simulink model "FG_costante_vs_filtro"  (R2020a)
settings: Solver=VariableStepAuto  StartTime=0.0  StopTime=10.0  RelTol=1e-3
values from neighbouring files (symbols this model uses):
  Aa = 2    [dati_tesi_modellosimulink.m]
  g = 9.81    [dati_tesi_modellosimulink.m]
  L = 0.3    [dati_tesi_modellosimulink.m]
  Lc = L/2    (= 0.15)    [dati_tesi_modellosimulink.m]
  M = 4    [dati_tesi_modellosimulink.m]
  mc = 0    [dati_tesi_modellosimulink.m]
  Ra = 1    [dati_tesi_modellosimulink.m]
  wb = 2*pi*2    (= 12.5663706144)    [dati_tesi_modellosimulink.m]
libraries: fuzblock x5, simulink x3, simulink_extras x2
settings Model: Creator=laura  LastModifiedBy=laura

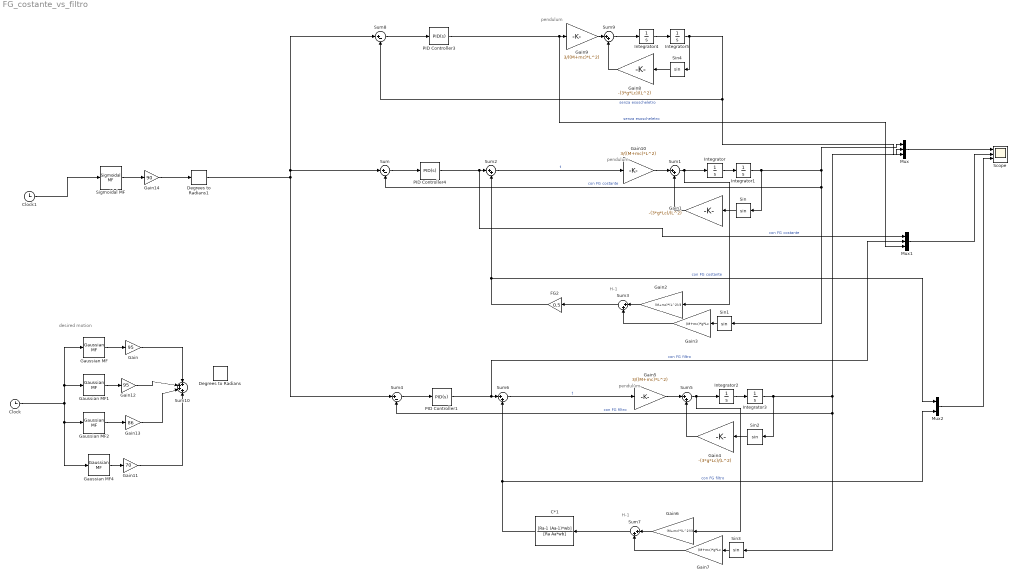
== system FG_costante_vs_filtro ==
  note: H-1
  note: pendulum
  note: pendulum
  note: H-1
  note: pendulum
  note: desired motion
  C*1 : TransferFcn  Numerator=[Ra-1 (Aa-1)*wb]  Denominator=[Ra Aa*wb]
  Clock : Clock
  Clock1 : Clock
  Degrees to Radians : simulink_extras/Transformations/Degrees to Radians
  Degrees to Radians1 : simulink_extras/Transformations/Degrees to Radians
  FG2 : Gain  Gain=0.5
  Gain : Gain  Gain=95
  Gain1 : Gain  Gain=-(3*g*Lc)/(L^2)
  Gain10 : Gain  Gain=3/((M+mc)*L^2)
  Gain11 : Gain  Gain=70
  Gain12 : Gain  Gain=95
  Gain13 : Gain  Gain=86
  Gain14 : Gain  Gain=90
  Gain2 : Gain  Gain=(M+mc)*(L^2)/3
  Gain3 : Gain  Gain=(M+mc)*g*Lc
  Gain4 : Gain  Gain=-(3*g*Lc)/(L^2)
  Gain5 : Gain  Gain=3/((M+mc)*L^2)
  Gain6 : Gain  Gain=(M+mc)*(L^2)/3
  Gain7 : Gain  Gain=(M+mc)*g*Lc
  Gain8 : Gain  Gain=-(3*g*Lc)/(L^2)
  Gain9 : Gain  Gain=3/((M+mc)*L^2)
  Gaussian MF : fuzblock/Membership  Functions/Gaussian MF  sigma=0.4  mu=1.78
      settings: SourceProductBaseCode=FL
  Gaussian MF1 : fuzblock/Membership  Functions/Gaussian MF  sigma=0.4  mu=7
      settings: SourceProductBaseCode=FL
  Gaussian MF2 : fuzblock/Membership  Functions/Gaussian MF  sigma=0.38  mu=3.42
      settings: SourceProductBaseCode=FL
  Gaussian MF4 : fuzblock/Membership  Functions/Gaussian MF  sigma=0.32  mu=2.63
      settings: SourceProductBaseCode=FL
  Integrator{,1..5} (6 alike) : Integrator
  Mux : Mux  Inputs=3
  Mux1 : Mux  Inputs=3
  Mux2 : Mux  Inputs=2
  PID Controller1 : simulink/Continuous/PID Controller  Controller=PID  Form=Parallel  TimeDomain=Continuous-time  UseExternalTs=off  SampleTime=-1  IntegratorMethod=Forward Euler  FilterMethod=Forward Euler  ControllerParametersSource=internal  P=20.396  I=105.7651  D=6.3413  UseFilter=on  N=150.7964  TunerSelectOption=Transfer Function Based (PID Tuner App)  InitialConditionSource=internal  InitialConditionForIntegrator=0  InitialConditionForFilter=0  DifferentiatorICPrevScaledInput=0  ExternalReset=none  TrackingMode=off  Kt=1  LimitOutput=off  UpperSaturationLimit=inf  LowerSaturationLimit=-inf  LinearizeAsGain=on  AntiWindupMode=none  Kb=1  POutMin=[]  POutMax=[]  IOutMin=[]  IOutMax=[]  DOutMin=[]  DOutMax=[]  NOutMin=[]  NOutMax=[]  SumOutMin=[]  SumOutMax=[]  SaturationOutMin=[]  SaturationOutMax=[]  PParamMin=[]  PParamMax=[]  IParamMin=[]  IParamMax=[]  DParamMin=[]  DParamMax=[]  NParamMin=[]  NParamMax=[]  KbParamMin=[]  KbParamMax=[]  KtParamMin=[]  KtParamMax=[]  KbOutMin=[]  KbOutMax=[]  KtOutMin=[]  KtOutMax=[]  IntegratorOutMin=[]  IntegratorOutMax=[]  FilterOutMin=[]  FilterOutMax=[]  SumI1OutMin=[]  SumI1OutMax=[]  SumI2OutMin=[]  SumI2OutMax=[]  SumI3OutMin=[]  SumI3OutMax=[]  SumI4OutMin=[]  SumI4OutMax=[]  SumDOutMin=[]  SumDOutMax=[]  DifferentiatorOutMin=[]  DifferentiatorOutMax=[]  FilterDiffOutCoefMin=[]  FilterDiffOutCoefMax=[]  ReciprocalOutMin=[]  ReciprocalOutMax=[]  SumDenOutMin=[]  SumDenOutMax=[]  SumNumOutMin=[]  SumNumOutMax=[]  DivideOutMin=[]  DivideOutMax=[]  UdiffTsProdOutMin=[]  UdiffTsProdOutMax=[]  NTsProdOutMin=[]  NTsProdOutMax=[]  UintegralTsProdOutMin=[]  UintegralTsProdOutMax=[]  UngainTsProdOutMin=[]  UngainTsProdOutMax=[]  IntegratorContinuousStateAttributes=''  IntegratorStateMustResolveToSignalObject=off  IntegratorRTWStateStorageClass=Auto  FilterContinuousStateAttributes=''  FilterStateMustResolveToSignalObject=off  FilterRTWStateStorageClass=Auto  ParallelPVariant=InternalParameters  IdealPVariant=Disabled  IVariant=InternalParameters  DVariant=InternalParameters  IntegratorVariant=Continuous  SatVariant=Disabled  AWVariant=Passthrough  PCopyVariant=Disabled  TRVariant=Disabled  FdbkBlocksVariant=Forward  IdealPFdbkVariant=Disabled  SatFdbkVariant=Disabled  DerivativeFilterVariant=ContFilter  NVariant=InternalParameters  NCopyVariant=Disabled  FilterICVariant=InternalICsFilter  IntegratorICVariant=InternalICs  ExternalResetVariant=Disabled  TRSumVariant=Passthrough  SumFdbkVariant=Disabled  SumVariant=Sum_PID  TsampFilterVariant=InternalTs  TsampNgainVariant=Passthrough  TsampIntegralVariant=Passthrough
  PID Controller3 : simulink/Continuous/PID Controller  Controller=PID  Form=Parallel  TimeDomain=Continuous-time  UseExternalTs=off  SampleTime=-1  IntegratorMethod=Forward Euler  FilterMethod=Forward Euler  ControllerParametersSource=internal  P=20.396  I=105.7651  D=6.3413  UseFilter=on  N=150.7964  TunerSelectOption=Transfer Function Based (PID Tuner App)  InitialConditionSource=internal  InitialConditionForIntegrator=0  InitialConditionForFilter=0  DifferentiatorICPrevScaledInput=0  ExternalReset=none  TrackingMode=off  Kt=1  LimitOutput=off  UpperSaturationLimit=inf  LowerSaturationLimit=-inf  LinearizeAsGain=on  AntiWindupMode=none  Kb=1  POutMin=[]  POutMax=[]  IOutMin=[]  IOutMax=[]  DOutMin=[]  DOutMax=[]  NOutMin=[]  NOutMax=[]  SumOutMin=[]  SumOutMax=[]  SaturationOutMin=[]  SaturationOutMax=[]  PParamMin=[]  PParamMax=[]  IParamMin=[]  IParamMax=[]  DParamMin=[]  DParamMax=[]  NParamMin=[]  NParamMax=[]  KbParamMin=[]  KbParamMax=[]  KtParamMin=[]  KtParamMax=[]  KbOutMin=[]  KbOutMax=[]  KtOutMin=[]  KtOutMax=[]  IntegratorOutMin=[]  IntegratorOutMax=[]  FilterOutMin=[]  FilterOutMax=[]  SumI1OutMin=[]  SumI1OutMax=[]  SumI2OutMin=[]  SumI2OutMax=[]  SumI3OutMin=[]  SumI3OutMax=[]  SumI4OutMin=[]  SumI4OutMax=[]  SumDOutMin=[]  SumDOutMax=[]  DifferentiatorOutMin=[]  DifferentiatorOutMax=[]  FilterDiffOutCoefMin=[]  FilterDiffOutCoefMax=[]  ReciprocalOutMin=[]  ReciprocalOutMax=[]  SumDenOutMin=[]  SumDenOutMax=[]  SumNumOutMin=[]  SumNumOutMax=[]  DivideOutMin=[]  DivideOutMax=[]  UdiffTsProdOutMin=[]  UdiffTsProdOutMax=[]  NTsProdOutMin=[]  NTsProdOutMax=[]  UintegralTsProdOutMin=[]  UintegralTsProdOutMax=[]  UngainTsProdOutMin=[]  UngainTsProdOutMax=[]  IntegratorContinuousStateAttributes=''  IntegratorStateMustResolveToSignalObject=off  IntegratorRTWStateStorageClass=Auto  FilterContinuousStateAttributes=''  FilterStateMustResolveToSignalObject=off  FilterRTWStateStorageClass=Auto  ParallelPVariant=InternalParameters  IdealPVariant=Disabled  IVariant=InternalParameters  DVariant=InternalParameters  IntegratorVariant=Continuous  SatVariant=Disabled  AWVariant=Passthrough  PCopyVariant=Disabled  TRVariant=Disabled  FdbkBlocksVariant=Forward  IdealPFdbkVariant=Disabled  SatFdbkVariant=Disabled  DerivativeFilterVariant=ContFilter  NVariant=InternalParameters  NCopyVariant=Disabled  FilterICVariant=InternalICsFilter  IntegratorICVariant=InternalICs  ExternalResetVariant=Disabled  TRSumVariant=Passthrough  SumFdbkVariant=Disabled  SumVariant=Sum_PID  TsampFilterVariant=InternalTs  TsampNgainVariant=Passthrough  TsampIntegralVariant=Passthrough
  PID Controller4 : simulink/Continuous/PID Controller  Controller=PID  Form=Parallel  TimeDomain=Continuous-time  UseExternalTs=off  SampleTime=-1  IntegratorMethod=Forward Euler  FilterMethod=Forward Euler  ControllerParametersSource=internal  P=20.396  I=105.7651  D=6.3413  UseFilter=on  N=150.7964  TunerSelectOption=Transfer Function Based (PID Tuner App)  InitialConditionSource=internal  InitialConditionForIntegrator=0  InitialConditionForFilter=0  DifferentiatorICPrevScaledInput=0  ExternalReset=none  TrackingMode=off  Kt=1  LimitOutput=off  UpperSaturationLimit=inf  LowerSaturationLimit=-inf  LinearizeAsGain=on  AntiWindupMode=none  Kb=1  POutMin=[]  POutMax=[]  IOutMin=[]  IOutMax=[]  DOutMin=[]  DOutMax=[]  NOutMin=[]  NOutMax=[]  SumOutMin=[]  SumOutMax=[]  SaturationOutMin=[]  SaturationOutMax=[]  PParamMin=[]  PParamMax=[]  IParamMin=[]  IParamMax=[]  DParamMin=[]  DParamMax=[]  NParamMin=[]  NParamMax=[]  KbParamMin=[]  KbParamMax=[]  KtParamMin=[]  KtParamMax=[]  KbOutMin=[]  KbOutMax=[]  KtOutMin=[]  KtOutMax=[]  IntegratorOutMin=[]  IntegratorOutMax=[]  FilterOutMin=[]  FilterOutMax=[]  SumI1OutMin=[]  SumI1OutMax=[]  SumI2OutMin=[]  SumI2OutMax=[]  SumI3OutMin=[]  SumI3OutMax=[]  SumI4OutMin=[]  SumI4OutMax=[]  SumDOutMin=[]  SumDOutMax=[]  DifferentiatorOutMin=[]  DifferentiatorOutMax=[]  FilterDiffOutCoefMin=[]  FilterDiffOutCoefMax=[]  ReciprocalOutMin=[]  ReciprocalOutMax=[]  SumDenOutMin=[]  SumDenOutMax=[]  SumNumOutMin=[]  SumNumOutMax=[]  DivideOutMin=[]  DivideOutMax=[]  UdiffTsProdOutMin=[]  UdiffTsProdOutMax=[]  NTsProdOutMin=[]  NTsProdOutMax=[]  UintegralTsProdOutMin=[]  UintegralTsProdOutMax=[]  UngainTsProdOutMin=[]  UngainTsProdOutMax=[]  IntegratorContinuousStateAttributes=''  IntegratorStateMustResolveToSignalObject=off  IntegratorRTWStateStorageClass=Auto  FilterContinuousStateAttributes=''  FilterStateMustResolveToSignalObject=off  FilterRTWStateStorageClass=Auto  ParallelPVariant=InternalParameters  IdealPVariant=Disabled  IVariant=InternalParameters  DVariant=InternalParameters  IntegratorVariant=Continuous  SatVariant=Disabled  AWVariant=Passthrough  PCopyVariant=Disabled  TRVariant=Disabled  FdbkBlocksVariant=Forward  IdealPFdbkVariant=Disabled  SatFdbkVariant=Disabled  DerivativeFilterVariant=ContFilter  NVariant=InternalParameters  NCopyVariant=Disabled  FilterICVariant=InternalICsFilter  IntegratorICVariant=InternalICs  ExternalResetVariant=Disabled  TRSumVariant=Passthrough  SumFdbkVariant=Disabled  SumVariant=Sum_PID  TsampFilterVariant=InternalTs  TsampNgainVariant=Passthrough  TsampIntegralVariant=Passthrough
  Scope : Scope  NumInputPorts=3
  Sigmoidal MF : fuzblock/Membership  Functions/Sigmoidal MF  a=4  c=5
      settings: SourceProductBaseCode=FL
  Sin{,1..4} (5 alike) : Trigonometry
  Sum : Sum  Inputs=|+-
  Sum{1..3,5..7,9} (7 alike) : Sum  Inputs=|++
  Sum10 : Sum  Inputs=++++
  Sum4 : Sum  Inputs=|+-
  Sum8 : Sum  Inputs=|+-
  wires:
  Sum8/1 -> PID Controller3/1
  Integrator4/1 -> Integrator5/1
  Sin1/1 -> Gain3/1
  Sin4/1 -> Gain8/1
  Integrator5/1 -> Mux/3, Sum8/2, Sin4/1  "senza esoscheletro"
  PID Controller3/1 -> Mux1/3, Gain9/1  "senza esoscheletro"
  Gain9/1 -> Sum9/1
  Gain1/1 -> Sum1/2
  Integrator/1 -> Integrator1/1
  Sum9/1 -> Integrator4/1
  Gain3/1 -> Sum3/2
  PID Controller4/1 -> Mux1/1, Sum2/1  "con FG costante"
  Sum3/1 -> FG2/1
  Sum2/1 -> Gain10/1  "t"
  Sum1/1 -> Integrator/1, Gain2/1
  Gain2/1 -> Sum3/1
  Gain8/1 -> Sum9/2
  Integrator1/1 -> Sin/1, Mux/1, Sin1/1, Sum/2  "con FG costante"
  FG2/1 -> Sum2/2, Mux2/1  "con FG costante"
  Sin/1 -> Gain1/1
  Sum/1 -> PID Controller4/1
  Gain10/1 -> Sum1/1
  Gain5/1 -> Sum5/1
  Degrees to Radians1/1 -> Sum4/1, Sum8/1, Sum/1
  Sin2/1 -> Gain4/1
  Sum4/1 -> PID Controller1/1
  Integrator3/1 -> Sin2/1, Mux/2, Sin3/1, Sum4/2  "con FG filtro"
  C*1/1 -> Mux2/2, Sum6/2  "con FG filtro"
  Gain6/1 -> Sum7/1
  Sum7/1 -> C*1/1
  PID Controller1/1 -> Mux1/2, Sum6/1  "con FG filtro"
  Sum5/1 -> Integrator2/1, Gain6/1
  Sum6/1 -> Gain5/1  "t"
  Integrator2/1 -> Integrator3/1
  Gain7/1 -> Sum7/2
  Gain4/1 -> Sum5/2
  Sin3/1 -> Gain7/1
  Mux/1 -> Scope/1
  Clock1/1 -> Sigmoidal MF/1
  Sigmoidal MF/1 -> Gain14/1
  Gaussian MF2/1 -> Gain13/1
  Gain13/1 -> Sum10/3
  Gain12/1 -> Sum10/2
  Gaussian MF/1 -> Gain/1
  Gain11/1 -> Sum10/4
  Gaussian MF1/1 -> Gain12/1
  Clock/1 -> Gaussian MF/1, Gaussian MF1/1, Gaussian MF4/1, Gaussian MF2/1
  Gain/1 -> Sum10/1
  Gaussian MF4/1 -> Gain11/1
  Mux1/1 -> Scope/2
  Mux2/1 -> Scope/3
  Gain14/1 -> Degrees to Radians1/1
